simulink model "RC_Circuit_low_pass_filter"  (R2022a)
settings: Solver=FixedStepAuto  StartTime=0.0  StopTime=10  FixedStep=0.001  RelTol=1e-3
model workspace (MAT data in the model file):
  R = [1 0.5]
libraries: simulink x1
settings Model: Creator=Kieran  LastModifiedBy=Kieran

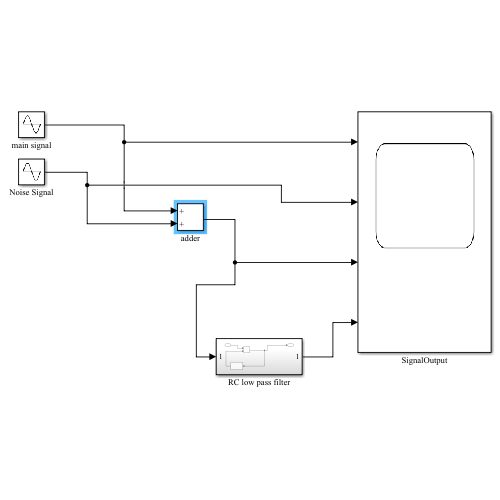
[thumbnail: Simulink's stored preview of the top-level diagram]
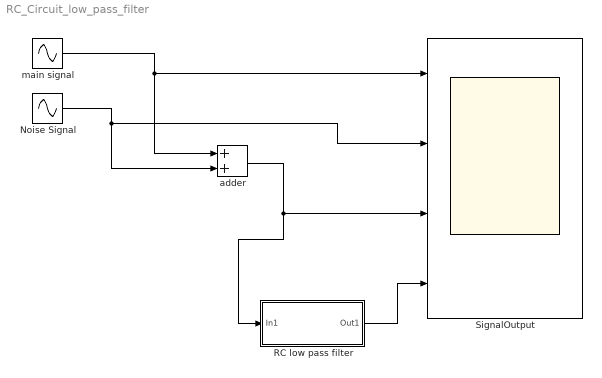
== system RC_Circuit_low_pass_filter ==
  Noise Signal : Sin  Amplitude=5  Frequency=10  SampleTime=0
  RC low pass filter : Subsystem
  SignalOutput : Scope  NumInputPorts=4
  adder : Sum
  main signal : Sin  Amplitude=50  SampleTime=0
  wires:
  main signal/1 -> adder/1, SignalOutput/1
  Noise Signal/1 -> adder/2, SignalOutput/2
  adder/1 -> RC low pass filter/1(In1), SignalOutput/3
  RC low pass filter/1(Out1) -> SignalOutput/4

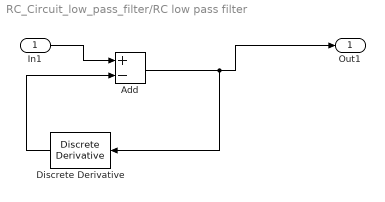
== system RC_Circuit_low_pass_filter/RC low pass filter ==
  In1 : Inport
  Add : Sum  Inputs=+-
  Discrete Derivative : simulink/Discrete/Discrete Derivative  gainval=1  ICPrevScaledInput=0.0  OutMin=[]  OutMax=[]  OutDataType=fixdt(1, 16)  OutScaling=2^-10  DoSatur=off
  Out1 : Outport
  wires:
  In1/1 -> Add/1
  Add/1 -> Discrete Derivative/1, Out1/1
  Discrete Derivative/1 -> Add/2
